simulink model "detumbling"  (R2021a)
settings: Solver=VariableStepAuto  StartTime=0.0  StopTime=15*Torb  RelTol=1e-3
libraries: sharedtransform x1, simulink_extras x1
settings Model: Creator=Laura  LastModifiedBy=Laura

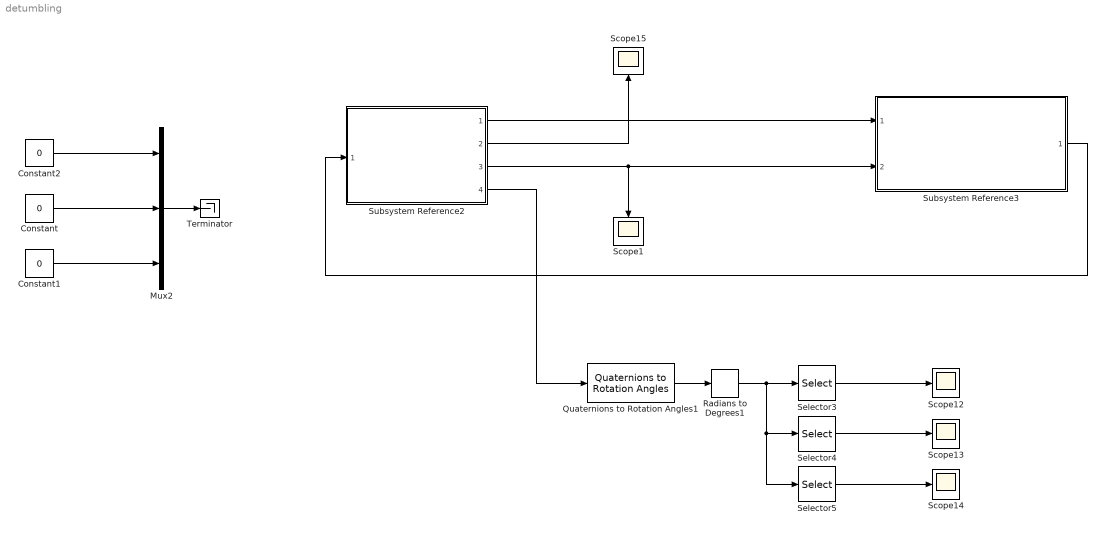
== system detumbling ==
  Constant : Constant  Value=0
  Constant1 : Constant  Value=0
  Constant2 : Constant  Value=0
  Mux2 : Mux  Inputs=3
  Quaternions to Rotation Angles1 : sharedtransform/Quaternions to Rotation Angles  rotationOrder=ZYX  aMode=aMode
      settings: SourceProductBaseCode=AE,PW,DR,MT,UV,VE
  Radians to Degrees1 : simulink_extras/Transformations/Radians to Degrees
  Scope{1,12..15} (5 alike) : Scope
  Selector3 : Selector  InputPortWidth=3  IndexOptions=Index vector (dialog)  Indices=[1]  OutputSizes=1
  Selector4 : Selector  InputPortWidth=3  IndexOptions=Index vector (dialog)  Indices=[2]  OutputSizes=1
  Selector5 : Selector  InputPortWidth=3  IndexOptions=Index vector (dialog)  Indices=[3]  OutputSizes=1
  Subsystem Reference2 : Subsystem  ReferencedSubsystem=DKE
  Subsystem Reference3 : Subsystem  ReferencedSubsystem=BdotController
  Terminator : Terminator
  wires:
  Constant/1 -> Mux2/2
  Constant1/1 -> Mux2/3
  Constant2/1 -> Mux2/1
  Quaternions to Rotation Angles1/1 -> Radians to Degrees1/1
  Radians to Degrees1/1 -> Selector5/1, Selector4/1, Selector3/1
  Selector3/1 -> Scope12/1
  Selector4/1 -> Scope13/1
  Selector5/1 -> Scope14/1
  Subsystem Reference2/4 -> Quaternions to Rotation Angles1/1
  Subsystem Reference2/1 -> Subsystem Reference3/1
  Subsystem Reference2/3 -> Subsystem Reference3/2, Scope1/1
  Subsystem Reference2/2 -> Scope15/1
  Subsystem Reference3/1 -> Subsystem Reference2/1
  Mux2/1 -> Terminator/1
